simulink model "FOG_v8"  (R2023b)
settings: Solver=FixedStepDiscrete  StartTime=0.0  StopTime=0.5  FixedStep=Ts_ctrl  RelTol=1e-3
undefined symbols (not defined in the file): a_act, a_meas, a_pi, b_act, b_meas, b_pi, Omega_controller_limit_deg_s, Omega_step_final, Omega_step_time, slope_per_deg_s, Ts_ctrl, wrap2pi_per_deg_s_Hz
settings Model: Creator=molik  LastModifiedBy=molik

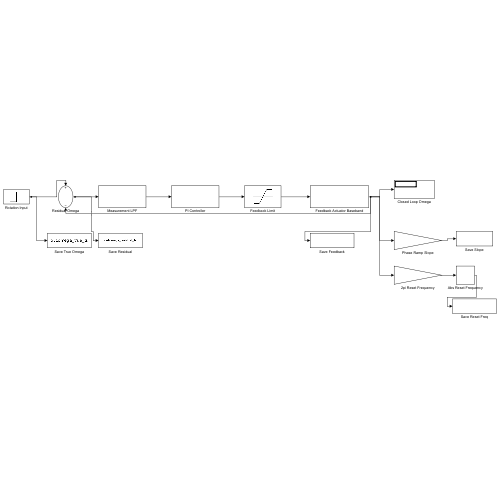
[thumbnail: Simulink's stored preview of the top-level diagram]
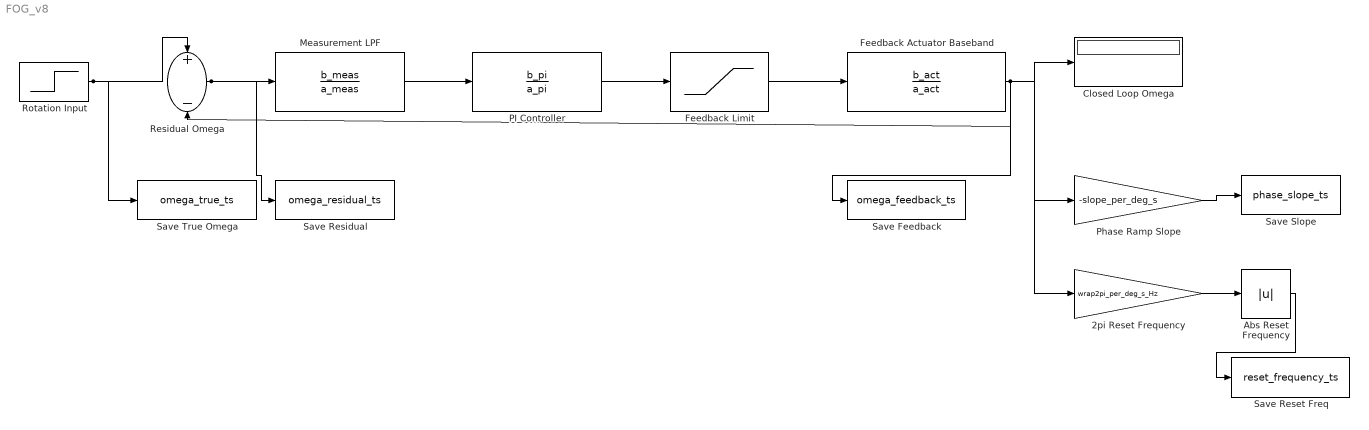
== system FOG_v8 ==
  2pi Reset Frequency : Gain  Gain=wrap2pi_per_deg_s_Hz
  Abs Reset Frequency : Abs  SaturateOnIntegerOverflow=off
  Closed Loop Omega : Display
  Feedback Actuator Baseband : DiscreteTransferFcn  Numerator=b_act  Denominator=a_act  SampleTime=Ts_ctrl
  Feedback Limit : Saturate  UpperLimit=Omega_controller_limit_deg_s  LowerLimit=-Omega_controller_limit_deg_s
  Measurement LPF : DiscreteTransferFcn  Numerator=b_meas  Denominator=a_meas  SampleTime=Ts_ctrl
  PI Controller : DiscreteTransferFcn  Numerator=b_pi  Denominator=a_pi  SampleTime=Ts_ctrl
  Phase Ramp Slope : Gain  Gain=-slope_per_deg_s
  Residual Omega : Sum  Inputs=+-
  Rotation Input : Step  Time=Omega_step_time  After=Omega_step_final  SampleTime=Ts_ctrl
  Save Feedback : ToWorkspace  VariableName=omega_feedback_ts  SaveFormat=Timeseries  SampleTime=-1
  Save Reset Freq : ToWorkspace  VariableName=reset_frequency_ts  SaveFormat=Timeseries  SampleTime=-1
  Save Residual : ToWorkspace  VariableName=omega_residual_ts  SaveFormat=Timeseries  SampleTime=-1
  Save Slope : ToWorkspace  VariableName=phase_slope_ts  SaveFormat=Timeseries  SampleTime=-1
  Save True Omega : ToWorkspace  VariableName=omega_true_ts  SaveFormat=Timeseries  SampleTime=-1
  wires:
  Rotation Input/1 -> Residual Omega/1, Save True Omega/1
  Residual Omega/1 -> Measurement LPF/1, Save Residual/1
  Measurement LPF/1 -> PI Controller/1
  PI Controller/1 -> Feedback Limit/1
  Feedback Limit/1 -> Feedback Actuator Baseband/1
  Feedback Actuator Baseband/1 -> Residual Omega/2, Closed Loop Omega/1, Save Feedback/1, Phase Ramp Slope/1, 2pi Reset Frequency/1
  Phase Ramp Slope/1 -> Save Slope/1
  2pi Reset Frequency/1 -> Abs Reset Frequency/1
  Abs Reset Frequency/1 -> Save Reset Freq/1
